simulink model "Test_timedelay"  (R2019a)
settings: Solver=FixedStepAuto  StartTime=0.0  StopTime=20  FixedStep=0.01  RelTol=1e-3
libraries: simulink x3
settings Model: Creator=huic  LastModifiedBy=huic

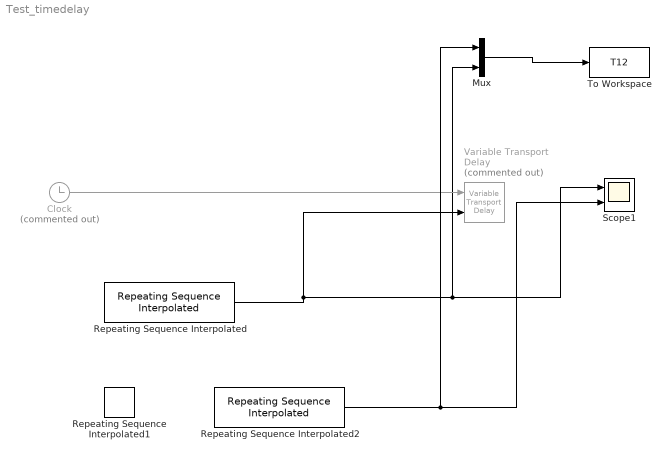
== system Test_timedelay ==
  Clock : Clock  Commented=on
  Mux : Mux  Inputs=2
  Repeating Sequence Interpolated : simulink/Sources/Repeating Sequence Interpolated  OutValues=[0 0 2 2.1 0.13 0.13 2.1 2.2 0.15].'  TimeValues=[0 2 4 8 10 12 14 18 20].'  LookUpMeth=Interpolation-Use End Values  tsamp=0.01  OutMin=[]  OutMax=[]  OutDataTypeStr=double  OutputDataTypeScalingMode=double  OutDataType=fixdt(0,8)  OutScaling=2^-10
  Repeating Sequence Interpolated1 : simulink/Sources/Repeating Sequence Interpolated  OutValues=[0 0 2 2.1 0.2].'  TimeValues=[0 2 4 8 10].'  LookUpMeth=Interpolation-Use End Values  tsamp=0.01  OutMin=[]  OutMax=[]  OutDataTypeStr=double  OutputDataTypeScalingMode=double  OutDataType=fixdt(0,8)  OutScaling=2^-10
  Repeating Sequence Interpolated2 : simulink/Sources/Repeating Sequence Interpolated  OutValues=[0 0 2 2 0.1 0].'  TimeValues=[0 2 4 8 9.8 10].'  LookUpMeth=Interpolation-Use End Values  tsamp=0.01  OutMin=[]  OutMax=[]  OutDataTypeStr=double  OutputDataTypeScalingMode=double  OutDataType=fixdt(0,8)  OutScaling=2^-10
  Scope1 : Scope  NumInputPorts=2
  To Workspace : ToWorkspace  VariableName=T12  SaveFormat=Structure With Time  SampleTime=-1
  Variable Transport Delay : VariableTransportDelay  Commented=on  MaximumDelay=10
  wires:
  Repeating Sequence Interpolated/1 -> Scope1/1, Mux/2, Variable Transport Delay/2
  Clock/1 -> Variable Transport Delay/1
  Repeating Sequence Interpolated2/1 -> Mux/1, Scope1/2
  Mux/1 -> To Workspace/1
